simulink library "ESTS_UOD_YawRateDifLatRef"  (R2022a)
settings: Solver=VariableStepAuto  StartTime=0.0  StopTime=10.0  RelTol=1e-3
settings Model: Creator=blatak  LastModifiedBy=blatak

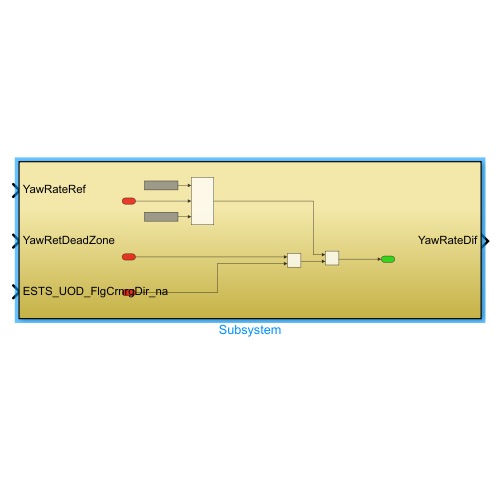
[thumbnail: Simulink's stored preview of the top-level diagram]
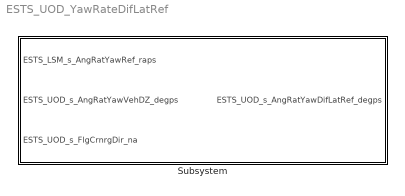
== system ESTS_UOD_YawRateDifLatRef ==
  Subsystem : Subsystem

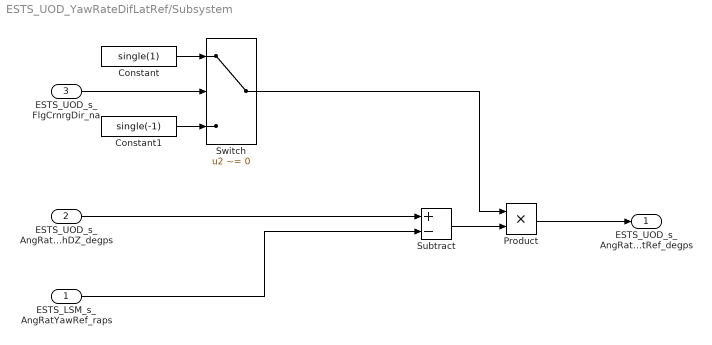
== system ESTS_UOD_YawRateDifLatRef/Subsystem ==
  ESTS_LSM_s_AngRatYawRef_raps : Inport
  ESTS_UOD_s_AngRatYawVehDZ_degps : Inport  Port=2
  ESTS_UOD_s_FlgCrnrgDir_na : Inport  Port=3
  Constant : Constant  Value=single(1)
  Constant1 : Constant  Value=single(-1)
  Product : Product
  Subtract : Sum  Inputs=+-
  Switch : Switch  Criteria=u2 ~= 0  SaturateOnIntegerOverflow=off  InputSameDT=off
  ESTS_UOD_s_AngRatYawDifLatRef_degps : Outport
  wires:
  Constant/1 -> Switch/1
  Switch/1 -> Product/1
  Product/1 -> ESTS_UOD_s_AngRatYawDifLatRef_degps/1
  ESTS_LSM_s_AngRatYawRef_raps/1 -> Subtract/2
  Constant1/1 -> Switch/3
  ESTS_UOD_s_FlgCrnrgDir_na/1 -> Switch/2
  Subtract/1 -> Product/2
  ESTS_UOD_s_AngRatYawVehDZ_degps/1 -> Subtract/1
